simulink model "test1_ACC"  (R2023a)
settings: Solver=FixedStepDiscrete  StartTime=0.0  StopTime=10.0  FixedStep=0.1  RelTol=1e-3  EnableMultiTasking=on
settings Model: Creator=Leo  LastModifiedBy=Leo
settings SolverCC: AlgebraicLoopSolver=TrustRegion  AutoInsertRateTranBlk=on
settings DataIOCC: LimitDataPoints=on
settings OptimizationCC: LifeSpan=inf
settings DebuggingCC: UnconnectedInputMsg=warning  UnconnectedOutputMsg=warning  UnconnectedLineMsg=warning  AllowSymbolicDim=off  SFUnexpectedBacktrackingDiag=warning  SFNoUnconditionalDefaultTransitionDiag=warning  SFExecutionAtInitializationDiag=none  ArithmeticOperatorsInVariantConditions=warning
settings ModelReferenceCC: EnableRefExpFcnMdlSchedulingChecks=on
settings SFSimCC: SimUseLocalCustomCode=off  CustomCodeUndefinedFunction=UseInterfaceOnly
settings RTWCC: RTWUseLocalCustomCode=off  DLArmComputeVersion=19.05
settings CodeAppCC: StateflowObjectComments=on
settings GRTTargetCC: TargetLangStandard=C89/C90 (ANSI)
settings ConfigComp: CovMetricSettings=dw  CovSaveCumulativeToWorkspaceVar=on  CovSaveSingleToWorkspaceVar=on  CovExternalEMLEnable=off

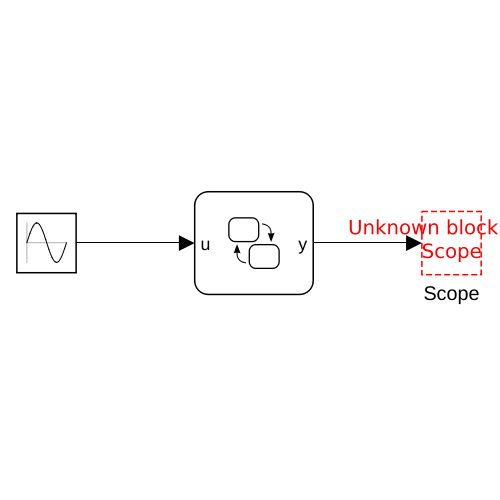
[thumbnail: Simulink's stored preview of the top-level diagram]
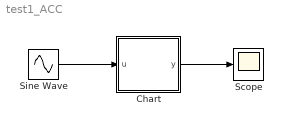
== system test1_ACC ==
  Chart : Stateflow chart  TreatAsAtomicUnit=on
  Scope : Scope
  Sine Wave : Sin  SampleTime=0
  wires:
  Sine Wave/1 -> Chart/1(u)
  Chart/1(y) -> Scope/1

== stateflow chart test1_ACC/Chart ==
  state ACC_OFF_MODE %State Name
    entry:
    Acceleration_mode = 0; % entry action
    % during:
  state ACC_STANDBY_MODE
    entry:
    Acceleration_Mode = 1;
  state ACC_ON_MODE
    state LeadVehicle_Detected_Follow
      entry:
      Acceleration_Mode  = 2;
    state LeadVehicle_Not_Detected
      entry:
      Acceleration_Mode  = 2;
    state LeadVehicle_Detected_Resume
      entry:
      Acceleration_Mode  = 3;
    state LeadVehicle_Not_Detected_Resume
      entry:
      Acceleration_Mode  = 1;
    state LeadVehicle_Speed_lessthen_Set_Speed
      entry:
      Acceleration_Mode  = 4;
    state LeadVehicle_Speed_Equal_Set_Speed
      entry:
      Acceleration_Mode  = 5;
    (default) -> LeadVehicle_Detected_Follow
    LeadVehicle_Speed_lessthen_Set_Speed -> LeadVehicle_Not_Detected
  (default) -> ACC_OFF_MODE %State Name
  ACC_OFF_MODE %State Name -> ACC_STANDBY_MODE : [CruiseSwitch==1]
      | % [transition condition]{action}
  ACC_STANDBY_MODE -> ACC_OFF_MODE %State Name : [CruiseSwitch==1]
  data: u input; y output
